simulink model "PD_LQR_VSC"  (R2024b)
settings: Solver=ode4  StartTime=0.0  StopTime=20  FixedStep=1e-3  RelTol=1e-3  EnableMultiTasking=on
values from neighbouring files (symbols this model uses):
  contr = listdlg(      'PromptString', 'Choose controller for the simulation:',      'SelectionMode', 'single',      'ListString', {'PD','LQR','MPC','off'},      'InitialValue', 1,      'Name', 'Controller Choice',      'ListSize', [300 70])    [MAIN.m]
  g = 9.81    [MAIN.m]
  i_steer = 15.4    [MAIN.m]
  Kd = 100    [MAIN.m]
  Kp = 20000    [MAIN.m]
  Kr_sched = K_sched(:,2)'    [MAIN.m]
  Kv_sched = K_sched(:,1)'    [MAIN.m]
  mu = 1    [MAIN.m]
  noise = 0    [MAIN.m]
  tau = 0.09    [MAIN.m]
  u_sched = linspace(60,100,N)/3.6    [MAIN.m]
  V_ref = 60/3.6    (= 16.6666666667)    [MAIN.m]
  wn = 11    [MAIN.m]
  xi = 0.7    [MAIN.m]
libraries: simulink x2
settings Model: Creator=bshyrokau  LastModifiedBy=nicvi
settings SolverCC: AlgebraicLoopSolver=TrustRegion
settings DataIOCC: SaveOutput=off  SignalLogging=off  DSMLogging=off  SaveTime=off  ReturnWorkspaceOutputs=off
settings OptimizationCC: ReuseModelBlockBuffer=off  LifeSpan=inf
settings DebuggingCC: UnconnectedInputMsg=warning  UnconnectedOutputMsg=warning  UnconnectedLineMsg=warning  AllowSymbolicDim=off  SFUnexpectedBacktrackingDiag=warning  SFNoUnconditionalDefaultTransitionDiag=warning  SFExecutionAtInitializationDiag=none  ArithmeticOperatorsInVariantConditions=warning
settings ModelReferenceCC: EnableRefExpFcnMdlSchedulingChecks=on  PropagateSignalLabelsOutOfModel=off
settings SFSimCC: SimUseLocalCustomCode=off  CustomCodeUndefinedFunction=UseInterfaceOnly
settings RTWCC: RTWUseLocalCustomCode=off  GPUComputeCapability=3.5  DLArmComputeVersion=19.05
settings CodeAppCC: StateflowObjectComments=on
settings GRTTargetCC: TargetLangStandard=C89/C90 (ANSI)
settings ConfigComp: CovMetricSettings=dw  CovSaveCumulativeToWorkspaceVar=on  CovSaveSingleToWorkspaceVar=on  CovExternalEMLEnable=off
settings SimscapeCC: SimscapeNormalizeSystem=off
settings ConfigurationSet: Description=SimMechanics 2G

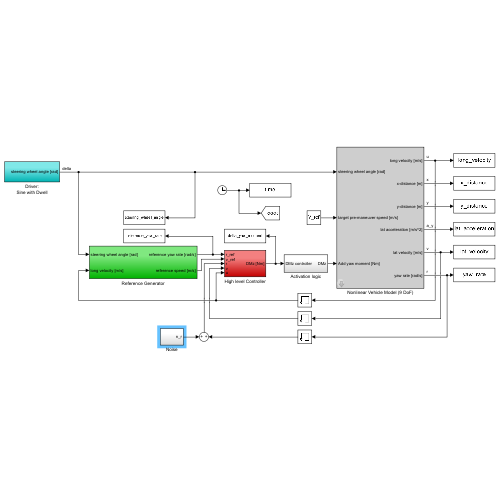
[thumbnail: Simulink's stored preview of the top-level diagram]
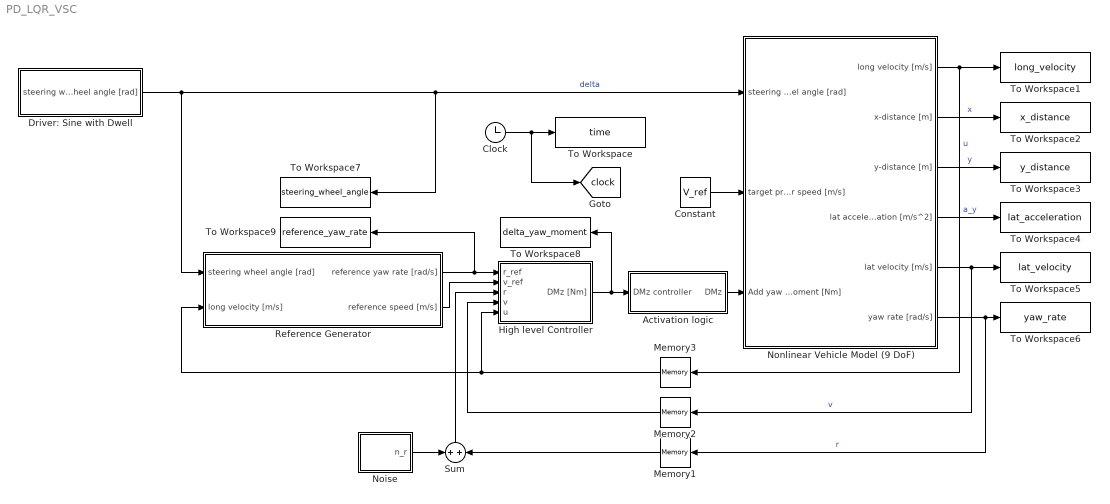
== system PD_LQR_VSC ==
  Activation logic : Subsystem
  Clock : Clock
  Constant : Constant  Value=V_ref
  Driver: Sine with Dwell : Subsystem
  High level Controller : Subsystem
  Memory1 : Memory
  Memory2 : Memory
  Memory3 : Memory
  Noise : Subsystem
  Nonlinear Vehicle Model (9 DoF) : Subsystem
      mask help: Simulink:masks:GenSFuncDesc_MD
      mask Help: eval('feval(''rtwprivate'',''rtwhelpview'',''rtw_sfcn_block'')');
  Reference Generator : Subsystem
  Sum : Sum  Inputs=+|+
  To Workspace : ToWorkspace  VariableName=time  SampleTime=-1
  To Workspace1 : ToWorkspace  VariableName=long_velocity  SampleTime=-1
  To Workspace2 : ToWorkspace  VariableName=x_distance  SampleTime=-1
  To Workspace3 : ToWorkspace  VariableName=y_distance  SampleTime=-1
  To Workspace4 : ToWorkspace  VariableName=lat_acceleration  SampleTime=-1
  To Workspace5 : ToWorkspace  VariableName=lat_velocity  SampleTime=-1
  To Workspace6 : ToWorkspace  VariableName=yaw_rate  SampleTime=-1
  To Workspace7 : ToWorkspace  VariableName=steering_wheel_angle  SampleTime=-1
  To Workspace8 : ToWorkspace  VariableName=delta_yaw_moment  SampleTime=-1
  To Workspace9 : ToWorkspace  VariableName=reference_yaw_rate  SampleTime=-1
  tag scope: clock=global
  wires:
  Driver: Sine with Dwell/1(steering wheel angle [rad]) -> Nonlinear Vehicle Model (9 DoF)/1(steering wheel angle [rad]), To Workspace7/1, Reference Generator/1(steering wheel angle [rad])  "delta"
  Reference Generator/1(reference yaw rate [rad/s]) -> To Workspace9/1, High level Controller/1(r_ref)
  High level Controller/1(DMz [Nm]) -> To Workspace8/1, Activation logic/1(DMz controller)
  Nonlinear Vehicle Model (9 DoF)/6(yaw rate [rad/s]) -> To Workspace6/1, Memory1/1  "r"
  Nonlinear Vehicle Model (9 DoF)/5(lat velocity [m/s]) -> To Workspace5/1, Memory2/1  "v"
  Nonlinear Vehicle Model (9 DoF)/1(long velocity [m/s]) -> To Workspace1/1, Memory3/1  "u"
  Nonlinear Vehicle Model (9 DoF)/4(lat acceleration [m/s^2]) -> To Workspace4/1  "a_y"
  Nonlinear Vehicle Model (9 DoF)/2(x-distance [m]) -> To Workspace2/1  "x"
  Nonlinear Vehicle Model (9 DoF)/3(y-distance [m]) -> To Workspace3/1  "y"
  Constant/1 -> Nonlinear Vehicle Model (9 DoF)/2(target pre-maneuver speed [m/s])
  Clock/1 -> To Workspace/1, [clock]
  Memory1/1 -> Sum/2
  Sum/1 -> High level Controller/3(r)
  Activation logic/1(DMz) -> Nonlinear Vehicle Model (9 DoF)/3(Add yaw moment [Nm])
  Noise/1(n_r) -> Sum/1
  Memory2/1 -> High level Controller/4(v)
  Memory3/1 -> High level Controller/5(u), Reference Generator/2(long velocity [m/s])
  Reference Generator/2(reference speed [m/s]) -> High level Controller/2(v_ref)

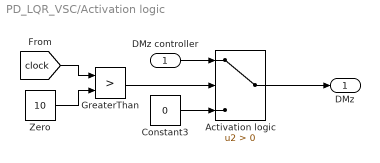
== system PD_LQR_VSC/Activation logic ==
  DMz controller : Inport
  Activation logic : Switch  Criteria=u2 > Threshold  SaturateOnIntegerOverflow=off  InputSameDT=off
  Constant3 : Constant  Value=0
  GreaterThan : RelationalOperator  Operator=>  OutDataTypeStr=boolean  RndMeth=Simplest  InputSameDT=off
  Zero : Constant  Value=10  OutDataTypeStr=Inherit: Inherit via back propagation
  DMz : Outport
  wires:
  [clock] -> GreaterThan/1
  GreaterThan/1 -> Activation logic/2
  Activation logic/1 -> DMz/1
  DMz controller/1 -> Activation logic/1
  Zero/1 -> GreaterThan/2
  Constant3/1 -> Activation logic/3

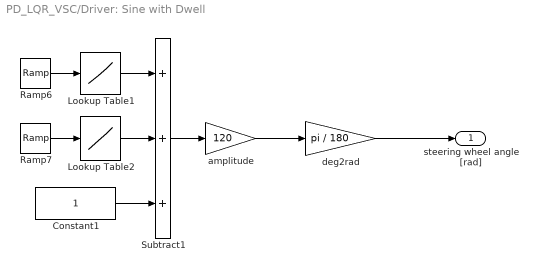
== system PD_LQR_VSC/Driver: Sine with Dwell ==
  Constant1 : Constant
  Lookup Table1 : Lookup  InputValues=[0:0.1:3*pi/2 3*pi/2+eps]*0.7  Table=sin([0:0.1:3*pi/2 3*pi/2+eps])  LookUpMeth=Interpolation-Use End Values  SaturateOnIntegerOverflow=off
  Lookup Table2 : Lookup  InputValues=[3*pi/2:0.1:2*pi 2*pi+eps]*0.7  Table=sin([3*pi/2:0.1:2*pi 2*pi+eps])  LookUpMeth=Interpolation-Use End Values  SaturateOnIntegerOverflow=off
  Ramp6 : simulink/Sources/Ramp  slope=pi  start=10  InitialOutput=0
  Ramp7 : simulink/Sources/Ramp  slope=pi  start=10+0.5  InitialOutput=0
  Subtract1 : Sum  Inputs=+++
  amplitude : Gain  Gain=120
  deg2rad : Gain  Gain=pi / 180
  steering wheel angle [rad] : Outport  VectorParamsAs1DForOutWhenUnconnected=off
  wires:
  Ramp6/1 -> Lookup Table1/1
  Ramp7/1 -> Lookup Table2/1
  Lookup Table2/1 -> Subtract1/2
  Lookup Table1/1 -> Subtract1/1
  Constant1/1 -> Subtract1/3
  Subtract1/1 -> amplitude/1
  amplitude/1 -> deg2rad/1
  deg2rad/1 -> steering wheel angle [rad]/1

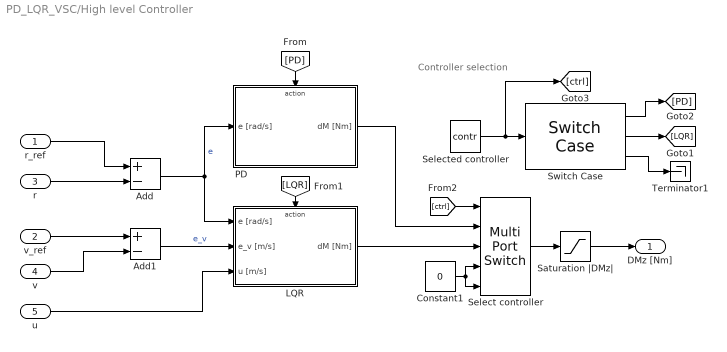
== system PD_LQR_VSC/High level Controller ==
  note: Controller selection
  r_ref : Inport
  v_ref : Inport  Port=2
  r : Inport  Port=3
  v : Inport  Port=4
  u : Inport  Port=5
  Add : Sum  Inputs=+-
  Add1 : Sum  Inputs=+-
  Constant1 : Constant  Value=0
  LQR : Subsystem
  PD : Subsystem
  Saturation |DMz| : Saturate  UpperLimit=10000  LowerLimit=-10000
  Select controller : MultiPortSwitch  Inputs=4  SaturateOnIntegerOverflow=off  InputSameDT=off
  Selected controller : Constant  Value=contr
  Switch Case : SwitchCase  CaseConditions={1,2,4}  ShowDefaultCase=off
  Terminator1 : Terminator
  DMz [Nm] : Outport  VectorParamsAs1DForOutWhenUnconnected=off
  wires:
  r_ref/1 -> Add/1
  Saturation |DMz|/1 -> DMz [Nm]/1
  PD/1(dM [Nm]) -> Select controller/2
  Add/1 -> PD/1(e [rad/s]), LQR/1(e [rad/s])  "e"
  r/1 -> Add/2
  v/1 -> Add1/2
  u/1 -> LQR/3(u [m/s])
  Select controller/1 -> Saturation |DMz|/1
  LQR/1(dM [Nm]) -> Select controller/3
  Selected controller/1 -> [ctrl], Switch Case/1
  Switch Case/1 -> [PD]
  Switch Case/2 -> [LQR]
  Switch Case/3 -> Terminator1/1
  [PD] -> PD/Action
  [LQR] -> LQR/Action
  [ctrl] -> Select controller/1
  v_ref/1 -> Add1/1
  Add1/1 -> LQR/2(e_v [m/s])  "e_v"
  Constant1/1 -> Select controller/4, Select controller/5

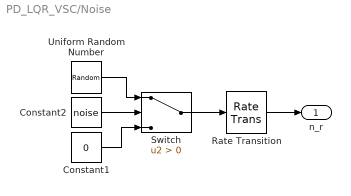
== system PD_LQR_VSC/Noise ==
  Constant1 : Constant  Value=0
  Constant2 : Constant  Value=noise
  Rate Transition : RateTransition
  Switch : Switch  Criteria=u2 > Threshold  SaturateOnIntegerOverflow=off  InputSameDT=off
  Uniform Random Number : UniformRandomNumber  Minimum=-deg2rad(0.5)  Maximum=deg2rad(0.5)  SampleTime=0.01
  n_r : Outport
  wires:
  Switch/1 -> Rate Transition/1
  Constant2/1 -> Switch/2
  Constant1/1 -> Switch/3
  Uniform Random Number/1 -> Switch/1
  Rate Transition/1 -> n_r/1

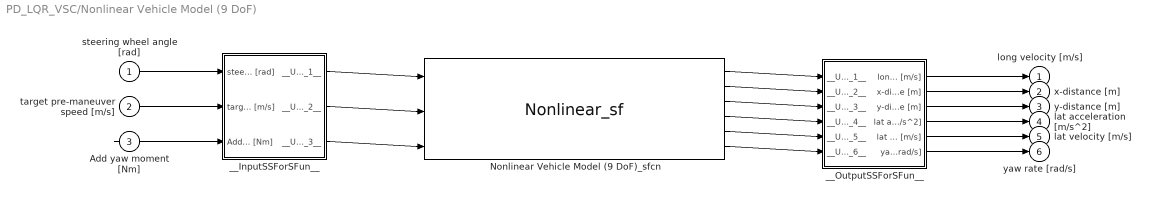
== system PD_LQR_VSC/Nonlinear Vehicle Model (9 DoF) ==
  steering wheel angle [rad] : Inport
  target pre-maneuver speed [m/s] : Inport  Port=2
  Add yaw moment [Nm] : Inport  Port=3
  Nonlinear Vehicle Model (9 DoF)_sfcn : S-Function  FunctionName=Nonlinear_sf  SFunctionModules=""  SFunctionDeploymentMode=off  EnableBusSupport=off  mask{rtw_sf_name=Nonlinear_sf, showVar=off}
      mask prompts: rtw_sf_name "Simulink:masks:GenSFuncName_MP"; showVar "Simulink:masks:GenSFuncShowModuleList_MP"
      mask help: Simulink:masks:GenSFuncDesc_MD
      mask init:
      | displist = '';
      | if ~strcmp(get_param(gcb, 'FunctionName'), rtw_sf_name);
      |   set_param(gcb, 'FunctionName', rtw_sf_name);
      | end
      | % Check if we are generating code
      | rtw_mode = false;
      | if strcmpi(get_param(bdroot(gcb),'SimulationStatus'),'Initializing')
      | 	rtw_mode = strcmpi(get_param(bdroot(gcb),'BuildingRTWCode'),'on') && ...
      | 		~strcmpi(get_param(bdroot(gcb),'TargetStyle'),'SimulationTarget');
      | end
      | if showVar || rtw_mode
      | 	if exist('rtwsfunc') == 2 | exist('rtwsfunc') == 6
      | 		tmplist = rtwsfunc(rtw_sf_name,gcb);
      | 		tmplist = DAStudio.message('Simulink:masks:GenSFuncListOfModules_IC', tmplist);
      | 	elseif showVar
      | 		tmplist1 = DAStudio.message('Simulink:masks:GenSFuncListOfModules_IC', '');
      |         tmplist2 = DAStudio.message('Simulink:masks:GenSFuncNotLicensed_IC');
      |         tmplist = [tmplist1 tmplist2];
      |  	end
      | end
      | if showVar
      |   displist = tmplist;
      | end
      settings: CopyFcn=|
      | if ~strcmp(get_param(gcb,'Linkstatus'),'none') && ...
      | ~strcmp(get_param(gcb,'Linkstatus'),'implicit')
      |   set_param(gcb,'LinkStatus','none');
      | end
      mask Help: eval('feval(''rtwprivate'',''rtwhelpview'',''rtw_sfcn_block'')');
      mask Display:
      | port_label('input',1,'steering wheel angle [rad]');
      | port_label('input',2,'target pre-maneuver speed [m/s]');
      | port_label('input',3,'Add yaw moment [Nm]');
      | port_label('output',1,'long velocity [m/s]');
      | port_label('output',2,'x-distance [m]');
      | port_label('output',3,'y-distance [m]');
      | port_label('output',4,'lat acceleration [m/s^2]');
      | port_label('output',5,'lat velocity [m/s]');
      | port_label('output',6,'yaw rate [rad/s]');
  __InputSSForSFun__ : Subsystem
  __OutputSSForSFun__ : Subsystem
  long velocity [m/s] : Outport  VectorParamsAs1DForOutWhenUnconnected=off
  x-distance [m] : Outport  Port=2  VectorParamsAs1DForOutWhenUnconnected=off
  y-distance [m] : Outport  Port=3  VectorParamsAs1DForOutWhenUnconnected=off
  lat acceleration [m/s^2] : Outport  Port=4  VectorParamsAs1DForOutWhenUnconnected=off
  lat velocity [m/s] : Outport  Port=5  VectorParamsAs1DForOutWhenUnconnected=off
  yaw rate [rad/s] : Outport  Port=6  VectorParamsAs1DForOutWhenUnconnected=off
  wires:
  steering wheel angle [rad]/1 -> __InputSSForSFun__/1(steering wheel angle [rad])
  target pre-maneuver speed [m/s]/1 -> __InputSSForSFun__/2(target pre-maneuver speed [m/s])
  Add yaw moment [Nm]/1 -> __InputSSForSFun__/3(Add yaw moment [Nm])
  __InputSSForSFun__/1(__UniqueOutportName__1__) -> Nonlinear Vehicle Model (9 DoF)_sfcn/1
  __InputSSForSFun__/2(__UniqueOutportName__2__) -> Nonlinear Vehicle Model (9 DoF)_sfcn/2
  __InputSSForSFun__/3(__UniqueOutportName__3__) -> Nonlinear Vehicle Model (9 DoF)_sfcn/3
  Nonlinear Vehicle Model (9 DoF)_sfcn/1 -> __OutputSSForSFun__/1(__UniqueInportName__1__)
  Nonlinear Vehicle Model (9 DoF)_sfcn/2 -> __OutputSSForSFun__/2(__UniqueInportName__2__)
  Nonlinear Vehicle Model (9 DoF)_sfcn/3 -> __OutputSSForSFun__/3(__UniqueInportName__3__)
  Nonlinear Vehicle Model (9 DoF)_sfcn/4 -> __OutputSSForSFun__/4(__UniqueInportName__4__)
  Nonlinear Vehicle Model (9 DoF)_sfcn/5 -> __OutputSSForSFun__/5(__UniqueInportName__5__)
  Nonlinear Vehicle Model (9 DoF)_sfcn/6 -> __OutputSSForSFun__/6(__UniqueInportName__6__)
  __OutputSSForSFun__/1(long velocity [m/s]) -> long velocity [m/s]/1
  __OutputSSForSFun__/2(x-distance [m]) -> x-distance [m]/1
  __OutputSSForSFun__/3(y-distance [m]) -> y-distance [m]/1
  __OutputSSForSFun__/4(lat acceleration [m/s^2]) -> lat acceleration [m/s^2]/1
  __OutputSSForSFun__/5(lat velocity [m/s]) -> lat velocity [m/s]/1
  __OutputSSForSFun__/6(yaw rate [rad/s]) -> yaw rate [rad/s]/1

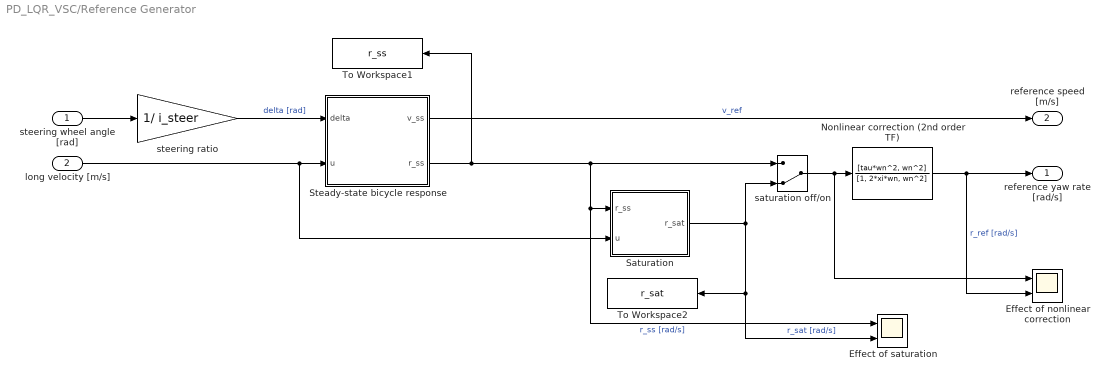
== system PD_LQR_VSC/Reference Generator ==
  steering wheel angle [rad] : Inport
  long velocity [m/s] : Inport  Port=2
  Effect of nonlinear correction : Scope  NumInputPorts=2
  Effect of saturation : Scope  NumInputPorts=2
  Nonlinear correction (2nd order TF) : TransferFcn  Numerator=[tau*wn^2, wn^2]  Denominator=[1, 2*xi*wn, wn^2]
  Saturation : Subsystem
  Steady-state bicycle response : MATLAB Function  TreatAsAtomicUnit=on
  To Workspace1 : ToWorkspace  VariableName=r_ss  SampleTime=-1
  To Workspace2 : ToWorkspace  VariableName=r_sat  SampleTime=-1
  saturation off/on : ManualSwitch  CurrentSetting=0
  steering ratio : Gain  Gain=1/ i_steer
  reference yaw rate [rad/s] : Outport  VectorParamsAs1DForOutWhenUnconnected=off
  reference speed [m/s] : Outport  Port=2  VectorParamsAs1DForOutWhenUnconnected=off
  wires:
  steering wheel angle [rad]/1 -> steering ratio/1
  steering ratio/1 -> Steady-state bicycle response/1(delta)  "delta [rad]"
  Nonlinear correction (2nd order TF)/1 -> Effect of nonlinear correction/2, reference yaw rate [rad/s]/1  "r_ref [rad/s]"
  Saturation/1(r_sat) -> Effect of saturation/2, To Workspace2/1, saturation off/on/2  "r_sat [rad/s]"
  long velocity [m/s]/1 -> Saturation/2(u), Steady-state bicycle response/2(u)
  Steady-state bicycle response/1(v_ss) -> reference speed [m/s]/1  "v_ref"
  Steady-state bicycle response/2(r_ss) -> saturation off/on/1, Effect of saturation/1, Saturation/1(r_ss), To Workspace1/1  "r_ss [rad/s]"
  saturation off/on/1 -> Effect of nonlinear correction/1, Nonlinear correction (2nd order TF)/1

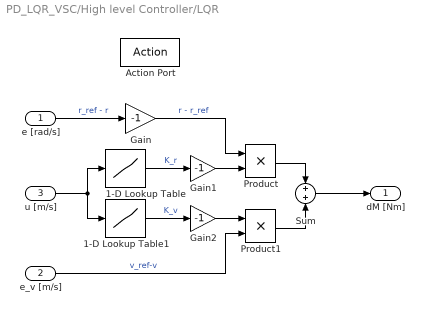
== system PD_LQR_VSC/High level Controller/LQR ==
  e [rad/s] : Inport
  e_v [m/s] : Inport  Port=2
  u [m/s] : Inport  Port=3
  Action Port : ActionPort  ActionPortLabel=case [ 2 ]:
  1-D Lookup Table : Lookup_n-D  NumberOfTableDimensions=1  BreakpointsForDimension1=u_sched  BreakpointsForDimension2=[1 8 27 64]  Table=Kr_sched  ExtrapMethod=Clip  UseLastTableValue=on  InternalRulePriority=Speed  RndMeth=Simplest
  1-D Lookup Table1 : Lookup_n-D  NumberOfTableDimensions=1  BreakpointsForDimension1=u_sched  BreakpointsForDimension2=[1 8 27 64]  Table=Kv_sched  ExtrapMethod=Clip  UseLastTableValue=on  InternalRulePriority=Speed  RndMeth=Simplest
  Gain : Gain  Gain=-1
  Gain1 : Gain  Gain=-1
  Gain2 : Gain  Gain=-1
  Product : Product
  Product1 : Product
  Sum : Sum  Inputs=+|+
  dM [Nm] : Outport
  wires:
  e [rad/s]/1 -> Gain/1  "r_ref - r"
  e_v [m/s]/1 -> Product1/2  "v_ref-v"
  Product/1 -> Sum/1
  Sum/1 -> dM [Nm]/1
  1-D Lookup Table/1 -> Gain1/1  "K_r"
  1-D Lookup Table1/1 -> Gain2/1  "K_v"
  u [m/s]/1 -> 1-D Lookup Table1/1, 1-D Lookup Table/1
  Gain/1 -> Product/1  "r - r_ref"
  Product1/1 -> Sum/2
  Gain1/1 -> Product/2
  Gain2/1 -> Product1/1

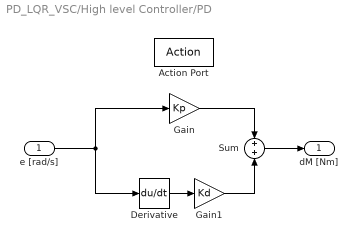
== system PD_LQR_VSC/High level Controller/PD ==
  e [rad/s] : Inport
  Action Port : ActionPort  ActionPortLabel=case [ 1 ]:
  Derivative : Derivative
  Gain : Gain  Gain=Kp
  Gain1 : Gain  Gain=Kd
  Sum : Sum  Inputs=+|+
  dM [Nm] : Outport
  wires:
  Sum/1 -> dM [Nm]/1
  Gain1/1 -> Sum/2
  Gain/1 -> Sum/1
  e [rad/s]/1 -> Derivative/1, Gain/1
  Derivative/1 -> Gain1/1

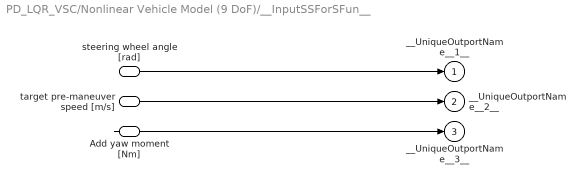
== system PD_LQR_VSC/Nonlinear Vehicle Model (9 DoF)/__InputSSForSFun__ ==
  steering wheel angle [rad] : Inport
  target pre-maneuver speed [m/s] : Inport  Port=2
  Add yaw moment [Nm] : Inport  Port=3
  __UniqueOutportName__1__ : Outport
  __UniqueOutportName__2__ : Outport  Port=2
  __UniqueOutportName__3__ : Outport  Port=3
  wires:
  steering wheel angle [rad]/1 -> __UniqueOutportName__1__/1
  target pre-maneuver speed [m/s]/1 -> __UniqueOutportName__2__/1
  Add yaw moment [Nm]/1 -> __UniqueOutportName__3__/1

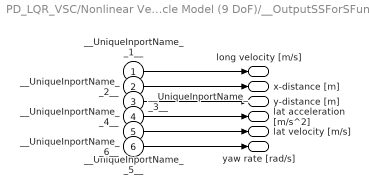
== system PD_LQR_VSC/Nonlinear Vehicle Model (9 DoF)/__OutputSSForSFun__ ==
  __UniqueInportName__1__ : Inport
  __UniqueInportName__2__ : Inport  Port=2
  __UniqueInportName__3__ : Inport  Port=3
  __UniqueInportName__4__ : Inport  Port=4
  __UniqueInportName__5__ : Inport  Port=5
  __UniqueInportName__6__ : Inport  Port=6
  long velocity [m/s] : Outport  VectorParamsAs1DForOutWhenUnconnected=off
  x-distance [m] : Outport  Port=2  VectorParamsAs1DForOutWhenUnconnected=off
  y-distance [m] : Outport  Port=3  VectorParamsAs1DForOutWhenUnconnected=off
  lat acceleration [m/s^2] : Outport  Port=4  VectorParamsAs1DForOutWhenUnconnected=off
  lat velocity [m/s] : Outport  Port=5  VectorParamsAs1DForOutWhenUnconnected=off
  yaw rate [rad/s] : Outport  Port=6  VectorParamsAs1DForOutWhenUnconnected=off
  wires:
  __UniqueInportName__1__/1 -> long velocity [m/s]/1
  __UniqueInportName__2__/1 -> x-distance [m]/1
  __UniqueInportName__3__/1 -> y-distance [m]/1
  __UniqueInportName__4__/1 -> lat acceleration [m/s^2]/1
  __UniqueInportName__5__/1 -> lat velocity [m/s]/1
  __UniqueInportName__6__/1 -> yaw rate [rad/s]/1

== system PD_LQR_VSC/Reference Generator/Saturation ==
  r_ss : Inport
  u : Inport  Port=2
  (avoid division by zero) : Subsystem
  compute r_max : Subsystem
  saturation : MATLAB Function  TreatAsAtomicUnit=on
  r_sat : Outport
  wires:
  compute r_max/1(r_max) -> saturation/2(r_max)
  saturation/1(r_sat) -> r_sat/1
  r_ss/1 -> saturation/1(r)
  u/1 -> (avoid division by zero)/1(In1)
  (avoid division by zero)/1(Out1) -> compute r_max/1(u)

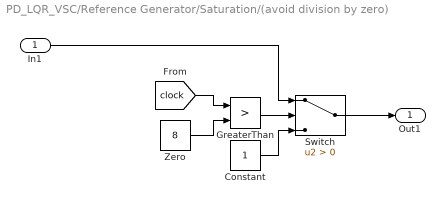
== system PD_LQR_VSC/Reference Generator/Saturation/(avoid division by zero) ==
  In1 : Inport
  Constant : Constant
  GreaterThan : RelationalOperator  Operator=>  OutDataTypeStr=boolean  RndMeth=Simplest  InputSameDT=off
  Switch : Switch  Criteria=u2 > Threshold  SaturateOnIntegerOverflow=off  InputSameDT=off
  Zero : Constant  Value=8  OutDataTypeStr=Inherit: Inherit via back propagation
  Out1 : Outport
  wires:
  Constant/1 -> Switch/3
  [clock] -> GreaterThan/1
  GreaterThan/1 -> Switch/2
  Switch/1 -> Out1/1
  In1/1 -> Switch/1
  Zero/1 -> GreaterThan/2

== system PD_LQR_VSC/Reference Generator/Saturation/compute r_max ==
  u : Inport
  Constant : Constant  Value=0.85*mu*g
  Divide : Product  Inputs=*/
  r_max : Outport
  wires:
  Constant/1 -> Divide/1
  Divide/1 -> r_max/1
  u/1 -> Divide/2

== matlab function PD_LQR_VSC/Reference Generator/Steady-state bicycle response ==
  data: v_ss output; delta input; u input; r_ss output
function [v_ss,r_ss]=ssBicycle(delta,u)

% Parameters
m = 1380;       % vehicle mass [Kg]    
L = 2.79;       % wheelbase [m]
lf = 1.384;     % distance from front axle to CoG [m]
lr = L-lf;      % distance from rear axle to CoG [m]
Caf = 120000;   % front axle cornering stiffness
Car = 190000;   % rear axle cornering stiffness
Iz = 2634.5;    % body inertia around z-axis [Kg m^2]

% Compute A matrix
A=zeros(2,2);
A(1,1)=-(Caf+Car)/(m*u);
A(1,2)=(lr*Car-lf*Caf)/(m*u)-u;
A(2,1)=(lr*Car-lf*Caf)/(Iz*u);
A(2,2)=-(lf^2*Caf+lr^2*Car)/(Iz*u);

% Compute B vector
B=[Caf/m Caf*lf/Iz]';

% Solve steady-state bicycle
x_ref=-A\(B*delta);
v_ss=x_ref(1);
r_ss=x_ref(2);

if any(isnan(x_ref))
    v_ss=0;
    r_ss=0;
end

end

== matlab function PD_LQR_VSC/Reference Generator/Saturation/saturation ==
  data: r input; r_sat output; r_max input
function r_sat=sat(r,r_max)

if r>r_max
    r_sat=r_max;
elseif r<-r_max
    r_sat=-r_max;
else
    r_sat=r;
end

end
